simulink model "ovencopy"  (R2020a)
settings: Solver=VariableStepAuto  StartTime=0.0  StopTime=10000  RelTol=1e-3
undefined symbols (not defined in the file): Cg, Cs, k, kc, kg, kr, sCon, Ta, u0
settings Model: Creator=tanzc  LastModifiedBy=tanzc
settings DataIOCC: SaveFormat=StructureWithTime  ReturnWorkspaceOutputs=off

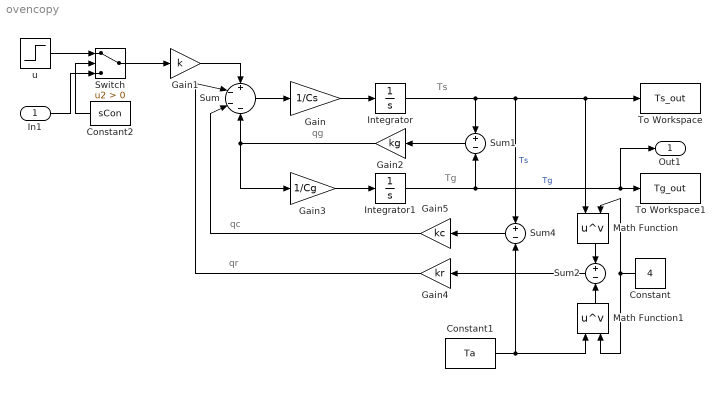
== system ovencopy ==
  note: Ts
  note: qg
  note: Tg
  note: qr
  note: qc
  In1 : Inport
  Constant : Constant  Value=4
  Constant1 : Constant  Value=Ta
  Constant2 : Constant  Value=sCon
  Gain : Gain  Gain=1/Cs
  Gain1 : Gain  Gain=k
  Gain2 : Gain  Gain=kg
  Gain3 : Gain  Gain=1/Cg
  Gain4 : Gain  Gain=kr
  Gain5 : Gain  Gain=kc
  Integrator : Integrator  Priority=1  InitialCondition=473.15
  Integrator1 : Integrator  Priority=2  InitialCondition=298.15
  Math Function : Math  Operator=pow  SignedPower=on  SaturateOnIntegerOverflow=on
  Math Function1 : Math  Operator=pow  SignedPower=on  SaturateOnIntegerOverflow=on
  Sum : Sum  Inputs=+---
  Sum1 : Sum  Inputs=+-
  Sum2 : Sum  Inputs=+-
  Sum4 : Sum  Inputs=+-
  Switch : Switch  Criteria=u2 > Threshold
  To Workspace : ToWorkspace  VariableName=Ts_out  SaveFormat=Structure With Time  SampleTime=-1
  To Workspace1 : ToWorkspace  VariableName=Tg_out  SaveFormat=Structure With Time  SampleTime=-1
  u : Step  Time=0  Before=u0  After=u0  SampleTime=0
  Out1 : Outport
  wires:
  Constant2/1 -> Switch/2
  Gain2/1 -> Gain3/1, Sum/4
  Constant1/1 -> Sum4/2, Math Function1/1
  Sum1/1 -> Gain2/1
  Switch/1 -> Gain1/1
  Sum2/1 -> Gain4/1
  Gain5/1 -> Sum/3
  Math Function1/1 -> Sum2/2
  Sum4/1 -> Gain5/1
  Gain4/1 -> Sum/2
  Gain3/1 -> Integrator1/1
  u/1 -> Switch/1
  Integrator1/1 -> Sum1/2, To Workspace1/1, Out1/1  "Tg"
  Constant/1 -> Math Function/2, Math Function1/2
  Integrator/1 -> Sum1/1, Sum4/1, Math Function/1, To Workspace/1  "Ts"
  Gain1/1 -> Sum/1
  In1/1 -> Switch/3
  Math Function/1 -> Sum2/1
  Gain/1 -> Integrator/1
  Sum/1 -> Gain/1
